simulink model "system_sim"  (R2015b)
settings: Solver=ode45  StartTime=0.0  StopTime=100  RelTol=1e-3
InitFcn:
  | param
undefined symbols (not defined in the file or in its folder): ctrl, P
settings Model: Creator=beard  LastModifiedBy=magiccjae
settings DataIOCC: SaveFormat=Array  SignalLoggingSaveFormat=ModelDataLogs
settings OptimizationCC: ExpressionDepthLimit=2147483647  InitFltsAndDblsToZero=on
settings DebuggingCC: UnderspecifiedInitializationDetection=Classic  MergeDetectMultiDrivingBlocksExec=none  SolverPrmCheckMsg=warning  FcnCallInpInsideContextMsg=UseLocalSettings  StateNameClashWarn=warning
settings HardwareCC: ProdBitPerPointer=32  ProdLargestAtomicFloat=None  ProdIntDivRoundTo=Undefined  ProdEndianess=Unspecified  ProdWordSize=32  ProdHWDeviceType=32-bit Generic
settings GRTTargetCC: GeneratePreprocessorConditionals=Disable all  CombineOutputUpdateFcns=off  GRTInterface=on
settings ConfigComp: CovModelRefEnable=Off

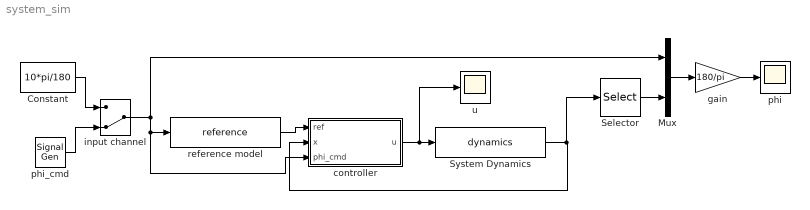
== system system_sim ==
  Constant : Constant  Value=10*pi/180
  Mux : Mux  Inputs=2
  Selector : Selector  InputPortWidth=2  IndexOptions=Index vector (dialog)  Indices=[1]  OutputSizes=1
  System Dynamics : S-Function  FunctionName=dynamics  Parameters=P  SFunctionDeploymentMode=off  EnableBusSupport=off
  controller : Subsystem
  gain : Gain  Gain=180/pi
  input channel : ManualSwitch  CurrentSetting=0
  phi : Scope
  phi_cmd : SignalGenerator  WaveForm=square  Amplitude=20*pi/180  Frequency=.05
  reference model : S-Function  FunctionName=reference  Parameters=P  SFunctionDeploymentMode=off  EnableBusSupport=off
  u : Scope
  wires:
  controller/1(u) -> u/1, System Dynamics/1
  System Dynamics/1 -> Selector/1, controller/2(x)
  Selector/1 -> Mux/2
  reference model/1 -> controller/1(ref)
  input channel/1 -> Mux/1, controller/3(phi_cmd), reference model/1
  Constant/1 -> input channel/1
  phi_cmd/1 -> input channel/2
  Mux/1 -> gain/1
  gain/1 -> phi/1

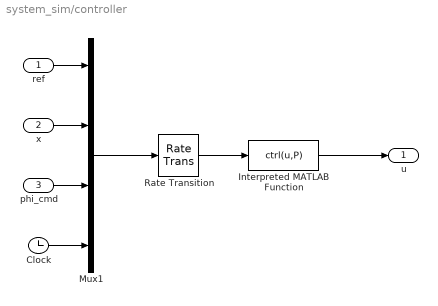
== system system_sim/controller ==
  ref : Inport
  x : Inport  Port=2
  phi_cmd : Inport  Port=3
  Clock : Clock
  Interpreted MATLAB Function : MATLABFcn  MATLABFcn=ctrl(u,P)  OutputDimensions=1
  Mux1 : Mux
  Rate Transition : RateTransition  OutPortSampleTime=P.Ts
  u : Outport
  wires:
  Mux1/1 -> Rate Transition/1
  ref/1 -> Mux1/1
  Interpreted MATLAB Function/1 -> u/1
  Rate Transition/1 -> Interpreted MATLAB Function/1
  x/1 -> Mux1/2
  Clock/1 -> Mux1/4
  phi_cmd/1 -> Mux1/3
